simulink model "vs_paper2002"  (R2018a)
settings: Solver=FixedStepAuto  StartTime=0.0  StopTime=15  FixedStep=ST  RelTol=1e-3
values from neighbouring files (symbols this model uses):
  k1 = 0.35    [paper2002.m]
  k2 = 0.01    [paper2002.m]
  k3 = 0.1    [paper2002.m]
  theta_0 = -0.3    [paper2002.m]
  x_0 = -3    [paper2002.m]
  x_ref = [0 0 0].'    [paper2002.m]
  y_0 = 0.1    [paper2002.m]
  y_th = 0.001    [paper2002.m]
settings Model: Creator=hkedw  LastModifiedBy=hkedw

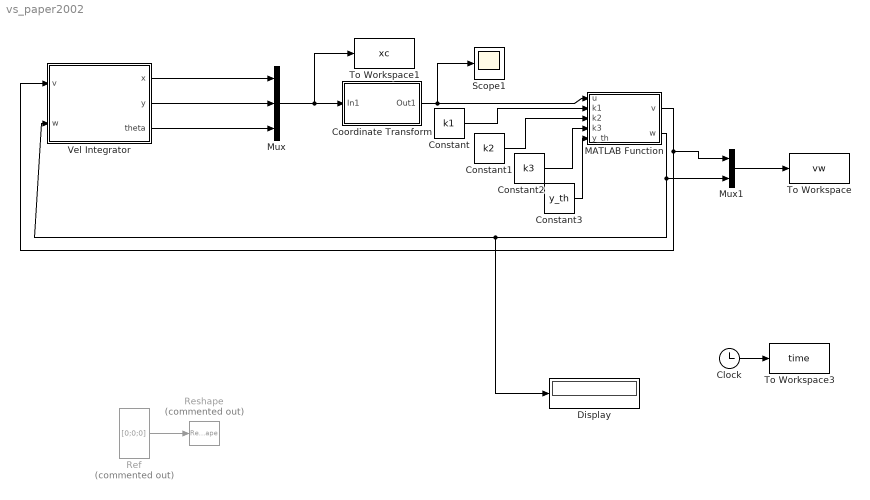
== system vs_paper2002 ==
  Clock : Clock
  Constant : Constant  Value=k1
  Constant1 : Constant  Value=k2
  Constant2 : Constant  Value=k3
  Constant3 : Constant  Value=y_th
  Coordinate Transform : Subsystem
  Display : Display
  MATLAB Function : MATLAB Function  TreatAsAtomicUnit=on
  Mux : Mux  Inputs=3
  Mux1 : Mux  Inputs=2
  Ref : Constant  Commented=on  Value=[0;0;0]  VectorParams1D=off
  Reshape : Reshape  Commented=on  OutputDimensionality=Column vector (2-D)
  Scope1 : Scope
  To Workspace : ToWorkspace  VariableName=vw  SaveFormat=Timeseries  SampleTime=-1
  To Workspace1 : ToWorkspace  VariableName=xc  SaveFormat=Timeseries  SampleTime=-1
  To Workspace3 : ToWorkspace  VariableName=time  SaveFormat=Timeseries  SampleTime=-1
  Vel Integrator : Subsystem
  wires:
  MATLAB Function/2(w) -> Mux1/2, Display/1, Vel Integrator/2(w)
  Vel Integrator/2(y) -> Mux/2
  Vel Integrator/3(theta) -> Mux/3
  Vel Integrator/1(x) -> Mux/1
  MATLAB Function/1(v) -> Mux1/1, Vel Integrator/1(v)
  Ref/1 -> Reshape/1
  Mux/1 -> To Workspace1/1, Coordinate Transform/1(In1)
  Constant/1 -> MATLAB Function/2(k1)
  Constant1/1 -> MATLAB Function/3(k2)
  Constant2/1 -> MATLAB Function/4(k3)
  Mux1/1 -> To Workspace/1
  Clock/1 -> To Workspace3/1
  Constant3/1 -> MATLAB Function/5(y_th)
  Coordinate Transform/1(Out1) -> Scope1/1, MATLAB Function/1(u)

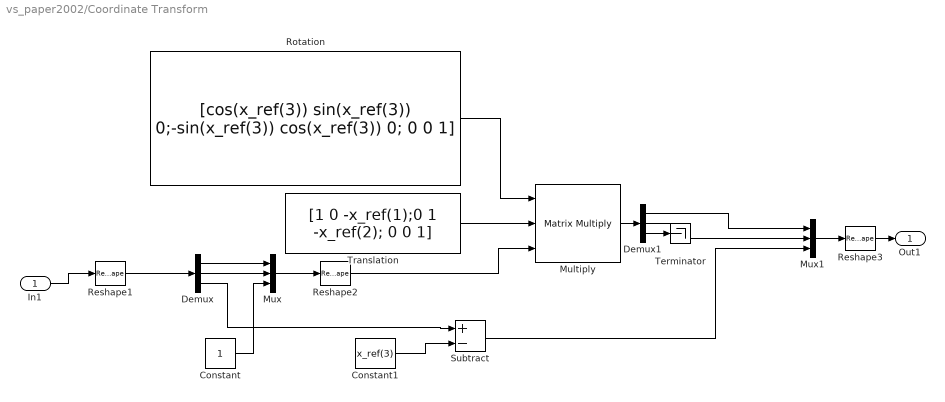
== system vs_paper2002/Coordinate Transform ==
  In1 : Inport
  Constant : Constant
  Constant1 : Constant  Value=x_ref(3)
  Demux : Demux  Outputs=3
  Demux1 : Demux  Outputs=3
  Multiply : Product  Inputs=3  Multiplication=Matrix(*)
  Mux : Mux  Inputs=3
  Mux1 : Mux  Inputs=3
  Reshape1 : Reshape  OutputDimensionality=Column vector (2-D)
  Reshape2 : Reshape  OutputDimensionality=Column vector (2-D)
  Reshape3 : Reshape  OutputDimensionality=Column vector (2-D)
  Rotation : Constant  Value=[cos(x_ref(3)) sin(x_ref(3)) 0;-sin(x_ref(3)) cos(x_ref(3)) 0; 0 0 1]  VectorParams1D=off
  Subtract : Sum  Inputs=+-
  Terminator : Terminator
  Translation : Constant  Value=[1 0 -x_ref(1);0 1 -x_ref(2); 0 0 1]  VectorParams1D=off
  Out1 : Outport
  wires:
  Demux1/1 -> Mux1/1
  Subtract/1 -> Mux1/3
  Reshape2/1 -> Multiply/3
  Demux1/3 -> Terminator/1
  Demux/2 -> Mux/2
  Reshape1/1 -> Demux/1
  Demux/1 -> Mux/1
  Constant/1 -> Mux/3
  Demux/3 -> Subtract/1
  Demux1/2 -> Mux1/2
  Mux/1 -> Reshape2/1
  Translation/1 -> Multiply/2
  Mux1/1 -> Reshape3/1
  Rotation/1 -> Multiply/1
  Constant1/1 -> Subtract/2
  Multiply/1 -> Demux1/1
  In1/1 -> Reshape1/1
  Reshape3/1 -> Out1/1

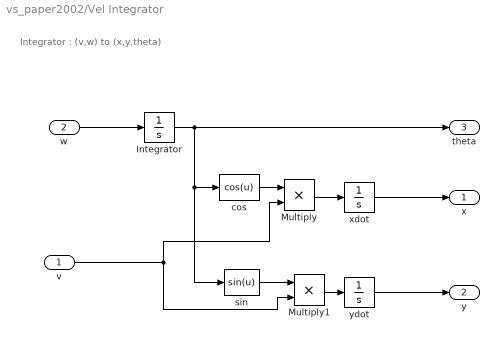
== system vs_paper2002/Vel Integrator ==
  note: Integrator : (v,w) to (x,y,theta)
  v : Inport
  w : Inport  Port=2
  Integrator : Integrator  InitialCondition=theta_0
  Multiply : Product
  Multiply1 : Product
  cos : MATLABFcn  MATLABFcn=cos(u)
  sin : MATLABFcn  MATLABFcn=sin(u)
  xdot : Integrator  InitialCondition=x_0
  ydot : Integrator  InitialCondition=y_0
  x : Outport
  y : Outport  Port=2
  theta : Outport  Port=3
  wires:
  w/1 -> Integrator/1
  Multiply/1 -> xdot/1
  cos/1 -> Multiply/1
  Multiply1/1 -> ydot/1
  ydot/1 -> y/1
  xdot/1 -> x/1
  sin/1 -> Multiply1/1
  Integrator/1 -> theta/1, sin/1, cos/1
  v/1 -> Multiply/2, Multiply1/2

== matlab function vs_paper2002/MATLAB Function ==
  data: u input; v output; k1 input; k2 input; k3 input; w output; y_th input
function [v,w] = fcn(u,k1,k2,k3,y_th)
c = u(3); % theta
x = u(1);
y = u(2);

if abs(y) > y_th
direct_judge = -cos(c)*x - sin(c)*y;

% need histerisis !!
if direct_judge == 0
    v = k3;
else
    v = sign(direct_judge)*k3;
end
w = -k2*c-k1*v*(sin(c)+0.0001)/(c+0.0001)*y;
else
    v = -x*k3;
    w = -k2*c-k1*v*(sin(c)+0.0001)/(c+0.0001)*y;
end
